simulink model "led_arduino"  (R2019a)
settings: Solver=FixedStepDiscrete  StartTime=0.0  StopTime=10  RelTol=1e-3
libraries: arduinolib x2
settings Model: FPTRunName=NoOverride  ExtModeTrigDuration=2  Creator=roslovetspv  LastModifiedBy=Pavel Roslovets
settings DataIOCC: ReturnWorkspaceOutputs=off
settings OptimizationCC: LifeSpan=1  MaxStackSize=64
settings DebuggingCC: SFUnexpectedBacktrackingDiag=warning  SFNoUnconditionalDefaultTransitionDiag=warning  SFExecutionAtInitializationDiag=none  ArithmeticOperatorsInVariantConditions=warning
settings HardwareCC: ProdBitPerInt=16  ProdBitPerPointer=16  ProdBitPerSizeT=16  ProdBitPerPtrDiffT=16  ProdLargestAtomicFloat=None  ProdWordSize=8  ProdHWDeviceType=Atmel->AVR
settings SFSimCC: SimUseLocalCustomCode=off  MATLABDynamicMemAlloc=off
settings RTWCC: SystemTargetFile=ert.tlc  HardwareBoard=Arduino Uno  TLCOptions=-aInlineSetEventsForThisBaseRateFcn=TLC_FALSE -aSuppressMultiTaskScheduler=TLC_FALSE -aRateBasedStepFcn=1  TemplateMakefile=ert_default_tmf  GenerateReport=on  RTWUseLocalCustomCode=off  Toolchain=Arduino AVR  BuildConfiguration=Faster Runs  IncludeHyperlinkInReport=on  LaunchReport=on  GenerateTraceInfo=on  GenerateTraceReport=on  GenerateTraceReportSl=on  GenerateTraceReportSf=on  GenerateTraceReportEml=on
settings CodeAppCC: ForceParamTrailComments=on  IgnoreCustomStorageClasses=off  OperatorAnnotations=on  SimulinkDataObjDesc=on  SFDataObjDesc=on  MATLABFcnDesc=on  InsertBlockDesc=on  StateflowObjectComments=on  MATLABSourceComments=on
settings ERTTargetCC: MultiwordLength=2048  SupportContinuousTime=on  SupportVariableSizeSignals=on
settings ConfigComp: CovMetricSettings=dw  CovHtmlReporting=on  CovSaveCumulativeToWorkspaceVar=on  CovSaveSingleToWorkspaceVar=on  CovExternalEMLEnable=off
settings SimscapeCC: SimscapeNormalizeSystem=off

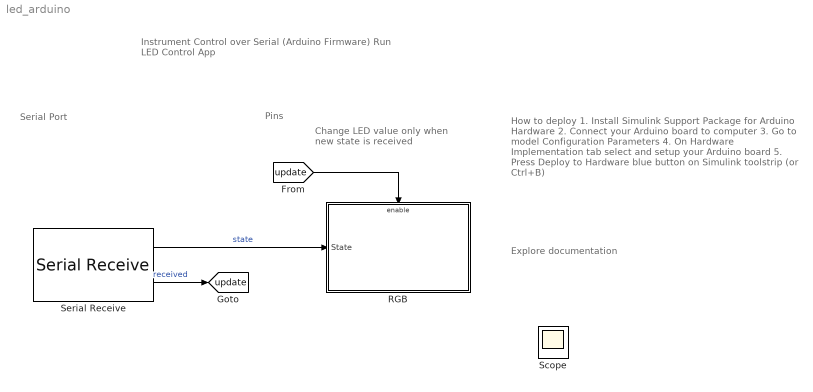
== system led_arduino ==
  note: Change LED value only when new state is received
  note: Explore documentation
  note: How to deploy
      | 1. Install Simulink Support Package for Arduino Hardware
      | 2. Connect your Arduino board to computer
      | 3. Go to model Configuration Parameters
      | 4. On Hardware Implementation tab select and setup your Arduino board
      | 5. Press Deploy to Hardware blue button on Simulink toolstrip (or Ctrl+B)
  note: Instrument Control over Serial
      | (Arduino Firmware)
      | Run LED Control App
  note: Pins
  note: Serial Port
  RGB : Subsystem  TreatAsAtomicUnit=on
  Serial Receive : arduinolib/Serial Receive  isARMArch=off  portNumber=0  DataType=uint8  Datalength=1  SampleTime=0.01  showOutStatus=on  blockPlatform=arduino
      settings: AttributesFormatString=Ts = %<SampleTime>  SourceProductName=Simulink Support Package for Arduino Hardware  SourceProductBaseCode=ARDUINO
  Scope : Scope
  tag scope: update=global
  wires:
  Serial Receive/1 -> RGB/1(State)  "state"
  Serial Receive/2 -> [update]  "received"
  [update] -> RGB/Enable

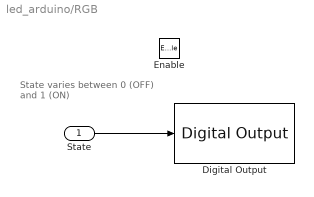
== system led_arduino/RGB ==
  note: State varies
      | between 0 (OFF) and 1 (ON)
  State : Inport  OutDataTypeStr=uint8
  Enable : EnablePort
  Digital Output : arduinolib/Digital Output  pinNumber=13  blockPlatform=arduino
  wires:
  State/1 -> Digital Output/1
